simulink model "lqg_cartpend_sim"  (R2016b)
settings: Solver=VariableStepAuto  StartTime=0.0  StopTime=50.0  RelTol=1e-3  EnableMultiTasking=on
values from neighbouring files (symbols this model uses):
  C = [1 0 0 0]    [lqg_simulinkINIT.m]    (also in lqg_simulinkINITBOOK.m)
  K = lqr(A,B,Q,R)    [lqg_simulinkINIT.m]    (also in lqg_simulinkINITBOOK.m)
  sysKF = ss(A-Kf*C,[B Kf],eye(4),0*[B Kf])    [lqg_simulinkINIT.m]    (also in lqg_simulinkINITBOOK.m)
  Vdmag = .04    (= 0.04)    [lqg_simulinkINITBOOK.m]
  Vn = .0000001    (= 1e-07)    [lqg_simulinkINIT.m]    (also in lqg_simulinkINITBOOK.m = 0.0002)
settings Model: Creator=sbrunton  LastModifiedBy=sbrunton
settings DataIOCC: LimitDataPoints=on
settings OptimizationCC: LifeSpan=inf
settings DebuggingCC: AllowSymbolicDim=off  SFUnexpectedBacktrackingDiag=warning  SFNoUnconditionalDefaultTransitionDiag=warning  SFExecutionAtInitializationDiag=none
settings ModelReferenceCC: PropagateSignalLabelsOutOfModel=off
settings GRTTargetCC: TargetLangStandard=C89/C90 (ANSI)
settings ConfigComp: CovMetricSettings=dw  CovHtmlReporting=on  CovSaveCumulativeToWorkspaceVar=on  CovSaveSingleToWorkspaceVar=on  CovExternalEMLEnable=off

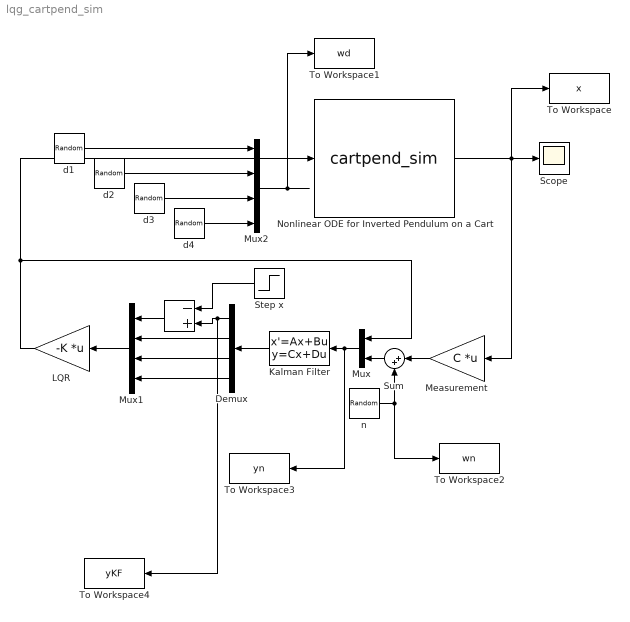
== system lqg_cartpend_sim ==
  " " : Sum  Inputs=-+
  Demux : Demux
  Kalman Filter : StateSpace  A=sysKF.a  B=sysKF.b  C=sysKF.c  D=sysKF.d  X0=[0 0 0 0]
  LQR : Gain  Tag=-Kr*xhat  Gain=-K  Multiplication=Matrix(K*u) (u vector)
  Measurement : Gain  Description=a  Gain=C  Multiplication=Matrix(K*u) (u vector)
  Mux : Mux  Inputs=2
  Mux1 : Mux
  Mux2 : Mux
  Nonlinear ODE for Inverted Pendulum on a Cart : S-Function  InitFcn=try, set_param(gcb,'FunctionName','cartpend_sim'), end  FunctionName=cartpend_sim  SFunctionModules=cartpend_sim_wrapper  SFunctionDeploymentMode=off  EnableBusSupport=off  mask(S-Function Builder){}
      mask help: Simulink:masks:SFunctionBuilder_MD
      mask init:
      | val = [[.9  0.75 0.75 1 1 .9 .9 1]',[1 1 0.75 0.75 .9 .9 1 .9]'];try , sys = get_param(gcb,'SfunBuilderFcnName');if isempty(sys), sys = get_param(gcb,'FunctionName'); end,catch, sys = get_param(gcb,'FunctionName'); end
      settings: CopyFcn=set_param(gcbh,'LinkStatus','none')  PreSaveFcn=try, set_param(gcb,'FunctionName','cartpend_sim'), end  OpenFcn=sfunctionwizard(gcbh)
      mask Display: plot(val(:,1),val(:,2)),disp(sys), port_label('input',1,'u'), port_label('input',2,'d'), port_label('output',1,'y')
  Scope : Scope
  Step x : Step  Time=10  SampleTime=0
  Sum : Sum  Inputs=|++
  To Workspace : ToWorkspace  VariableName=x  SaveFormat=Timeseries  SampleTime=-1
  To Workspace1 : ToWorkspace  VariableName=wd  SaveFormat=Timeseries  SampleTime=-1
  To Workspace2 : ToWorkspace  VariableName=wn  SaveFormat=Timeseries  SampleTime=-1
  To Workspace3 : ToWorkspace  VariableName=yn  SaveFormat=Timeseries  SampleTime=-1
  To Workspace4 : ToWorkspace  VariableName=yKF  SaveFormat=Timeseries  SampleTime=-1
  d1 : RandomNumber  Variance=Vdmag
  d2 : RandomNumber  Variance=Vdmag  Seed=1
  d3 : RandomNumber  Variance=Vdmag  Seed=2
  d4 : RandomNumber  Variance=Vdmag  Seed=3
  n : RandomNumber  Variance=Vn  Seed=4
  wires:
  LQR/1 -> Mux/1, Nonlinear ODE for Inverted Pendulum on a Cart/1
  Nonlinear ODE for Inverted Pendulum on a Cart/1 -> To Workspace/1, Measurement/1, Scope/1
  Mux/1 -> To Workspace3/1, Kalman Filter/1
  Demux/2 -> Mux1/2
  Demux/4 -> Mux1/4
  Mux1/1 -> LQR/1
  " "/1 -> Mux1/1
  Kalman Filter/1 -> Demux/1
  d1/1 -> Mux2/1
  d4/1 -> Mux2/4
  d2/1 -> Mux2/2
  d3/1 -> Mux2/3
  Sum/1 -> Mux/2
  Measurement/1 -> Sum/1
  n/1 -> To Workspace2/1, Sum/2
  Demux/3 -> Mux1/3
  Step x/1 -> " "/1
  Mux2/1 -> To Workspace1/1
  Demux/1 -> To Workspace4/1, " "/2
